simulink model "AirTestHarness"  (R2024a)
settings: configuration reference "standardSILConfiguraitonParams" (kept outside this file)
settings Model: Creator=gdela  LastModifiedBy=jerem
settings ConfigSetRef: SourceName=standardSILConfiguraitonParams  SourceLocation=Base Workspace

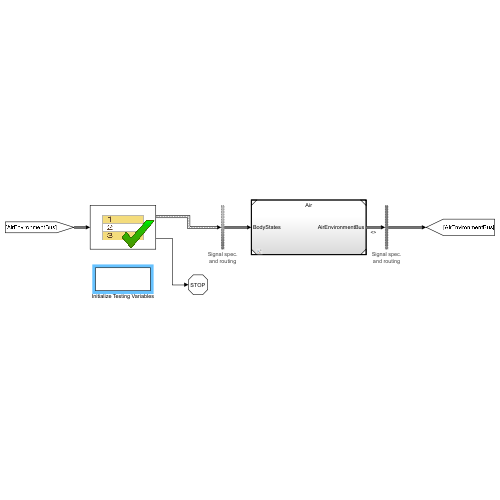
[thumbnail: Simulink's stored preview of the top-level diagram]
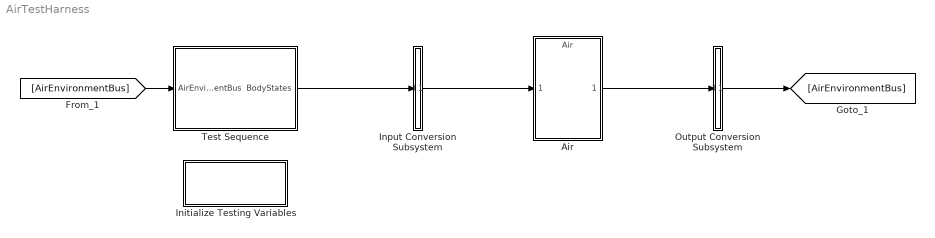
== system AirTestHarness ==
  Air : ModelReference  ModelNameDialog=Air  SimulationMode=Normal  ModelReferenceVersion=1.36
  Initialize Testing Variables : Subsystem
      settings: OpenFcn=AirTestHarnessInit
  Input Conversion Subsystem : Subsystem  Tag=__SLT_ICS__  Description=|
      | Signal spec.
      | and routing
      settings: AttributesFormatString=%<Description>
  Output Conversion Subsystem : Subsystem  Tag=__SLT_OCS__  Description=|
      | Signal spec.
      | and routing
      mask init:
      | ICDictionary = get_param(bdroot, 'DataDictionary');
      | if isempty(ICDictionary)
      |    ICScope = Simulink.data.BaseWorkspace;
      | else
      |    ICScope = Simulink.data.DataDictionary(ICDictionary);
      | end
      | 
      | IC1 = Simulink.Bus.createMATLABStruct('AirEnvironmentBus', [], [1 1], ICScope);
      settings: AttributesFormatString=%<Description>
  Test Sequence : Test Sequence  TreatAsAtomicUnit=on
  wires:
  Test Sequence/1(BodyStates) -> Input Conversion Subsystem/1(Inport_1)
  [AirEnvironmentBus] -> Test Sequence/1(AirEnvironmentBus)
  Output Conversion Subsystem/1(Outport_1) -> [AirEnvironmentBus]
  Air/1 -> Output Conversion Subsystem/1(Inport_1)
  Input Conversion Subsystem/1(Outport_1) -> Air/1

== system AirTestHarness/Initialize Testing Variables ==

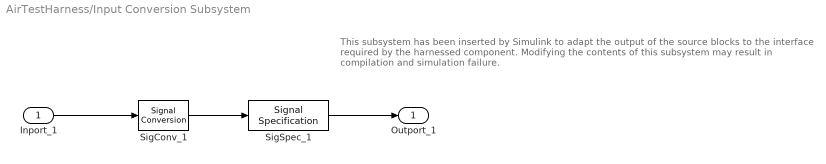
== system AirTestHarness/Input Conversion Subsystem ==
  note: This subsystem has been inserted by Simulink to adapt the output of the source blocks to the interface required by the harnessed component.
      |  Modifying the contents of this subsystem may result in compilation and simulation failure.
  Inport_1 : Inport
  SigConv_1 : SignalConversion  ConversionOutput=Virtual bus  OverrideOpt=off
  SigSpec_1 : SignalSpecification  OutDataTypeStr=Bus: BodyStateBus  SampleTime=[-1, 0]
  Outport_1 : Outport
  wires:
  SigSpec_1/1 -> Outport_1/1
  SigConv_1/1 -> SigSpec_1/1
  Inport_1/1 -> SigConv_1/1

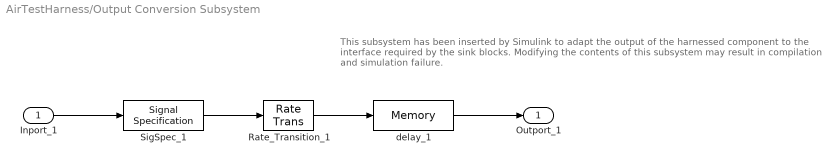
== system AirTestHarness/Output Conversion Subsystem ==
  note: This subsystem has been inserted by Simulink to adapt the output of the harnessed component to the interface required by the sink blocks.
      |  Modifying the contents of this subsystem may result in compilation and simulation failure.
  Inport_1 : Inport
  Rate_Transition_1 : RateTransition  OutPortSampleTimeOpt=Inherit
  SigSpec_1 : SignalSpecification  OutDataTypeStr=Bus: AirEnvironmentBus  Dimensions=[1]
  delay_1 : Memory  InitialCondition=IC1
  Outport_1 : Outport
  wires:
  Inport_1/1 -> SigSpec_1/1
  SigSpec_1/1 -> Rate_Transition_1/1
  Rate_Transition_1/1 -> delay_1/1
  delay_1/1 -> Outport_1/1

== stateflow chart AirTestHarness/Test Sequence ==
  state Scenario_1
    state Initialize
      %% Initialize data outputs.
      stopTest = false;
      BodyStates.aircraftVelInNED_mps = zeros(3,1);
      BodyStates.aircraftPosInNED_m = zeros(3,1);
      BodyStates.aircraftEulerAngles_rad = zeros(3,1);
      BodyStates.aircraftVelInBody_mps = zeros(3,1);
      BodyStates.aircraftAngVelInBody_radps = zeros(3,1);
      BodyStates.aircraftAngAccelInBody_radps2 = zeros(3,1);
      BodyStates.aircraftAccelInBody_mps2 = zeros(3,1);
      BodyStates.DCM_be = zeros(3,3);
    state Test1
      % AirTestHarnessInit.m defines workspace parameters
      % This test simply ensures that AirEnvironmentBus outputs are connected correctly
      verify(isClose(AirEnvironmentBus.windSpeedInNED_mps(1), 4));
      verify(isClose(AirEnvironmentBus.windSpeedInNED_mps(2), 3));
      verify(isClose(AirEnvironmentBus.windSpeedInNED_mps(3), 2));
      verify(isClose(AirEnvironmentBus.airTemperature_K, 288.15));
      verify(isClose(AirEnvironmentBus.airPressure_Pa, 1.01325e5));
      verify(isClose(AirEnvironmentBus.airDensity_kgpm3, 1.225));
      verify(isClose(AirEnvironmentBus.speedOfSound_mps, 340.29412435));
    state EndTest
      stopTest = true;
    (default) -> Initialize
    Initialize -> Test1 : [
        | after(3,sec)
        | ]
    Test1 -> EndTest : [
        | true
        | ]
  (default) -> Scenario_1 : {assert(Active_Scenario_Index == 1,'The value of Scenario Parameter ''Active_Scenario_Index'' is not valid. Use the index of the scenario to specify it.')}
  data: AirEnvironmentBus input Bus: AirEnvironmentBus size=[1]; BodyStates output Bus: BodyStateBus size=[1]; Active_Scenario_Index parameter =1; stopTest output
